simulink model "req17"  (R2019a)
settings: Solver=FixedStepAuto  StartTime=0.0  StopTime=100  RelTol=1e-3
libraries: simulink x4
settings Model: Creator=e40014285  LastModifiedBy=e40014285
settings ConfigComp: CovScope=ReferencedModels  CovHTMLOptions=-sRT=1 -sVT=0 -aTS=1 -bRG=1 -bTC=1 -hTR=0 -nFC=0 -nFD=1 -scm=1 -bcm=1 -xEv=0 -xEM=0  CovHtmlReporting=on  CovCumulativeReport=on  DVMaxProcessTime=6000  DVModelCoverageObjectives=EnhancedMCDC  DVTestSuiteOptimization=Auto  DVDetectOutOfBounds=on  DVReportPDFFormat=on  DVRebuildModelRepresentation=Always

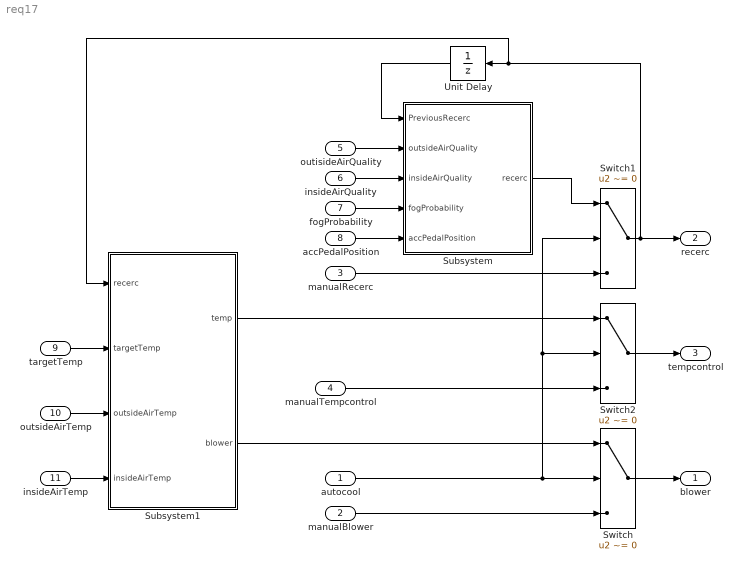
== system req17 ==
  autocool : Inport
  manualBlower : Inport  Port=2
  manualRecerc : Inport  Port=3
  manualTempcontrol : Inport  Port=4
  outisideAirQuality : Inport  Port=5
  insideAirQuality : Inport  Port=6
  fogProbability : Inport  Port=7
  accPedalPosition : Inport  Port=8
  targetTemp : Inport  Port=9
  outsideAirTemp : Inport  Port=10
  insideAirTemp : Inport  Port=11
  Subsystem : Subsystem
  Subsystem1 : Subsystem
  Switch : Switch  Criteria=u2 ~= 0
  Switch1 : Switch  Criteria=u2 ~= 0
  Switch2 : Switch  Criteria=u2 ~= 0
  Unit Delay : UnitDelay  SampleTime=-1  HasFrameUpgradeWarning=on
  blower : Outport
  recerc : Outport  Port=2
  tempcontrol : Outport  Port=3
  wires:
  autocool/1 -> Switch1/2, Switch2/2, Switch/2
  manualBlower/1 -> Switch/3
  Switch/1 -> blower/1
  manualRecerc/1 -> Switch1/3
  Switch1/1 -> recerc/1, Subsystem1/1(recerc), Unit Delay/1
  Switch2/1 -> tempcontrol/1
  manualTempcontrol/1 -> Switch2/3
  Unit Delay/1 -> Subsystem/1(PreviousRecerc)
  Subsystem/1(recerc) -> Switch1/1
  outisideAirQuality/1 -> Subsystem/2(outsideAirQuality)
  insideAirQuality/1 -> Subsystem/3(insideAirQuality)
  fogProbability/1 -> Subsystem/4(fogProbability)
  accPedalPosition/1 -> Subsystem/5(accPedalPosition)
  Subsystem1/2(blower) -> Switch/1
  Subsystem1/1(temp) -> Switch2/1
  targetTemp/1 -> Subsystem1/2(targetTemp)
  outsideAirTemp/1 -> Subsystem1/3(outsideAirTemp)
  insideAirTemp/1 -> Subsystem1/4(insideAirTemp)

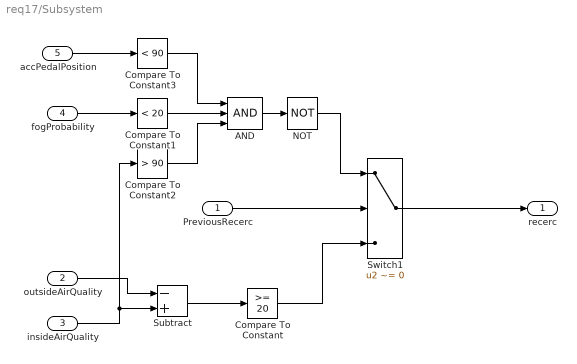
== system req17/Subsystem ==
  PreviousRecerc : Inport
  outsideAirQuality : Inport  Port=2
  insideAirQuality : Inport  Port=3
  fogProbability : Inport  Port=4
  accPedalPosition : Inport  Port=5
  AND : Logic  Inputs=3  AllPortsSameDT=off  OutDataTypeStr=boolean
  Compare To Constant : simulink/Logic and Bit Operations/Compare To Constant  relop=>=  const=20  OutDataTypeStr=boolean
  Compare To Constant1 : simulink/Logic and Bit Operations/Compare To Constant  relop=<  const=20  OutDataTypeStr=boolean
  Compare To Constant2 : simulink/Logic and Bit Operations/Compare To Constant  relop=>  const=90  OutDataTypeStr=boolean
  Compare To Constant3 : simulink/Logic and Bit Operations/Compare To Constant  relop=<  const=90  OutDataTypeStr=boolean
  NOT : Logic  Operator=NOT  AllPortsSameDT=off  OutDataTypeStr=boolean
  Subtract : Sum  Inputs=-+
  Switch1 : Switch  Criteria=u2 ~= 0
  recerc : Outport
  wires:
  PreviousRecerc/1 -> Switch1/2
  outsideAirQuality/1 -> Subtract/1
  insideAirQuality/1 -> Compare To Constant2/1, Subtract/2
  Subtract/1 -> Compare To Constant/1
  Compare To Constant/1 -> Switch1/3
  Switch1/1 -> recerc/1
  fogProbability/1 -> Compare To Constant1/1
  accPedalPosition/1 -> Compare To Constant3/1
  Compare To Constant3/1 -> AND/1
  Compare To Constant1/1 -> AND/2
  Compare To Constant2/1 -> AND/3
  AND/1 -> NOT/1
  NOT/1 -> Switch1/1

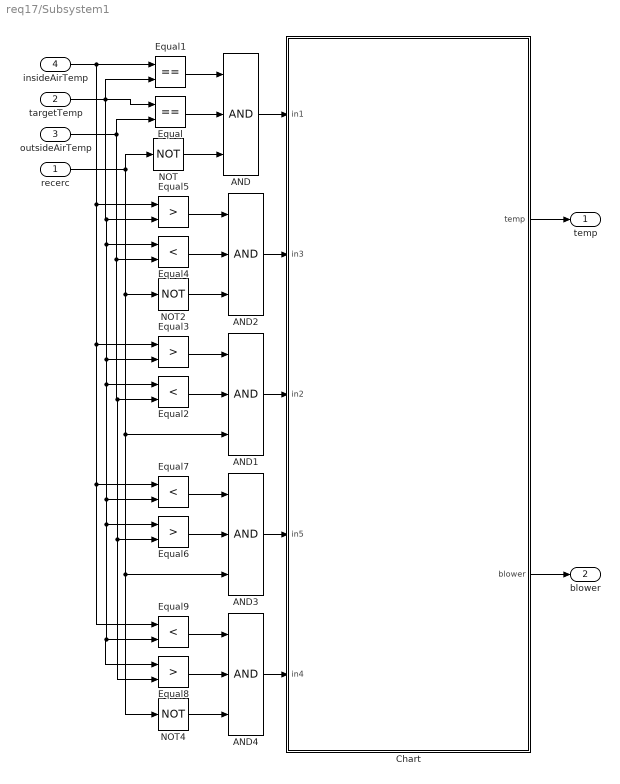
== system req17/Subsystem1 ==
  recerc : Inport
  targetTemp : Inport  Port=2
  outsideAirTemp : Inport  Port=3
  insideAirTemp : Inport  Port=4
  AND{,1..4} (5 alike) : Logic  Inputs=3  AllPortsSameDT=off  OutDataTypeStr=boolean
  Chart : Stateflow chart  BlockKeywords=__PRM__SERIALIZED__DATA__:Stateflow Chart,Stateflow Diagram  TreatAsAtomicUnit=on
  Equal : RelationalOperator  Operator===  OutDataTypeStr=boolean  RndMeth=Simplest
  Equal1 : RelationalOperator  Operator===  OutDataTypeStr=boolean  RndMeth=Simplest
  Equal{2,4,7,9} (4 alike) : RelationalOperator  Operator=<  OutDataTypeStr=boolean  RndMeth=Simplest
  Equal{3,5..6,8} (4 alike) : RelationalOperator  Operator=>  OutDataTypeStr=boolean  RndMeth=Simplest
  NOT : Logic  Operator=NOT  AllPortsSameDT=off  OutDataTypeStr=boolean
  NOT2 : Logic  Operator=NOT  AllPortsSameDT=off  OutDataTypeStr=boolean
  NOT4 : Logic  Operator=NOT  AllPortsSameDT=off  OutDataTypeStr=boolean
  temp : Outport
  blower : Outport  Port=2
  wires:
  Chart/1(temp) -> temp/1
  Equal/1 -> AND/2
  Chart/2(blower) -> blower/1
  AND/1 -> Chart/1(in1)
  NOT/1 -> AND/3
  Equal1/1 -> AND/1
  outsideAirTemp/1 -> Equal6/2, Equal8/2, Equal2/2, Equal4/2, Equal/2
  Equal3/1 -> AND1/1
  Equal2/1 -> AND1/2
  targetTemp/1 -> Equal/1, Equal1/2, Equal5/2, Equal4/1, Equal3/2, Equal2/1, Equal7/2, Equal6/1, Equal9/2, Equal8/1
  insideAirTemp/1 -> Equal7/1, Equal9/1, Equal3/1, Equal5/1, Equal1/1
  AND1/1 -> Chart/3(in2)
  NOT2/1 -> AND2/3
  Equal4/1 -> AND2/2
  Equal5/1 -> AND2/1
  AND2/1 -> Chart/2(in3)
  Equal7/1 -> AND3/1
  Equal6/1 -> AND3/2
  recerc/1 -> AND1/3, AND3/3, NOT4/1, NOT2/1, NOT/1
  AND3/1 -> Chart/4(in5)
  Equal9/1 -> AND4/1
  Equal8/1 -> AND4/2
  NOT4/1 -> AND4/3
  AND4/1 -> Chart/5(in4)

== stateflow chart req17/Subsystem1/Chart ==
  state state1
    blower=2;
    temp=50;
  state transition
  state state2
    blower=3;
    temp=0
  state state3
    blower=1;
    temp=0
  state state4
    blower=1;
    temp=100
  state state5
    blower=3;
    temp=100
  (default) -> state1
  transition -> state1 [order 1] : [in1]
  state1 -> transition : [in2||in3||in4||in5]
  transition -> state2 [order 2] : [in2]
  state2 -> transition : [in1||in3||in4||in5]
  transition -> state3 [order 3] : [in3]
  state3 -> transition : [in1||in2||in4||in5]
  transition -> state4 [order 4] : [in4]
  state4 -> transition : [in1||in2||in3||in5]
  transition -> state5 [order 5] : [in5]
  state5 -> transition : [in1||in2||in3||in4]
  data: in1 input; in3 input; in2 input; in5 input; in4 input; temp output; blower output
